simulink model "FMtestHarness"  (R2024b)
settings: Solver=VariableStepAuto  StartTime=0.0  StopTime=10.0  RelTol=1e-3  AbsTol=1e-3
model workspace: external: MAT-File VehicleharnessData.mat (data not in the file)
values from neighbouring files (symbols this model uses):
  VehicleHarn =     [VehicleharnessData.mat]
settings Model: DataDictionary=VTOLDynamicsData.sldd  Creator=saprasad  LastModifiedBy=jjha
settings SolverCC: AutoScaleAbsTol=off  AlgebraicLoopSolver=TrustRegion  MaxZcPerStep=1
settings DebuggingCC: UnconnectedInputMsg=warning  UnconnectedOutputMsg=warning  UnconnectedLineMsg=warning  SymbolicDimsDataTypeCodeGenerationDiagnostic=none
settings ModelReferenceCC: EnableRefExpFcnMdlSchedulingChecks=on
settings SFSimCC: CustomCodeUndefinedFunction=UseInterfaceOnly
settings RTWCC: GPUComputeCapability=3.5  DLArmComputeVersion=19.05
settings SimscapeCC: SimscapeLogType=all  SimscapeLogSimulationStatistics=on  SimscapeLogDataHistory=10000

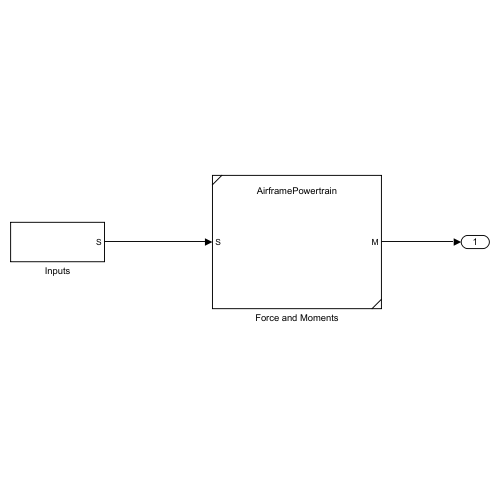
[thumbnail: Simulink's stored preview of the top-level diagram]
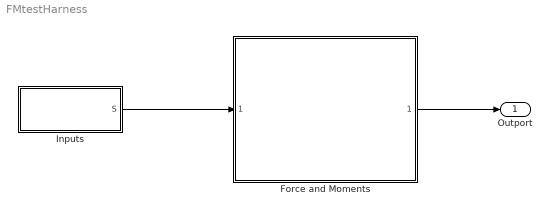
== system FMtestHarness ==
  Force and Moments : Subsystem  ReferencedSubsystem=AirframePowertrain
  Inputs : Subsystem
  Outport : Outport
  wires:
  Force and Moments/1 -> Outport/1
  Inputs/1(S) -> Force and Moments/1

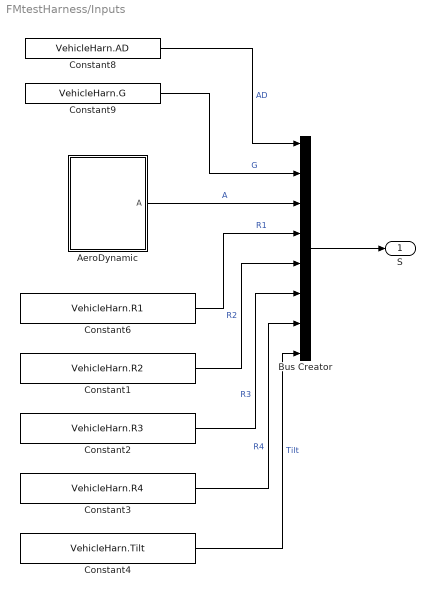
== system FMtestHarness/Inputs ==
  AeroDynamic : Subsystem
  Bus Creator : BusCreator  Inputs=8
  Constant1 : Constant  Value=VehicleHarn.R2  OutDataTypeStr=Bus: Vehicle_R2
  Constant2 : Constant  Value=VehicleHarn.R3  OutDataTypeStr=Bus: Vehicle_R3
  Constant3 : Constant  Value=VehicleHarn.R4  OutDataTypeStr=Bus: Vehicle_R4
  Constant4 : Constant  Value=VehicleHarn.Tilt  OutDataTypeStr=Bus: Vehicle_Tilt
  Constant6 : Constant  Value=VehicleHarn.R1  OutDataTypeStr=Bus: Vehicle_R1
  Constant8 : Constant  Value=VehicleHarn.AD  OutDataTypeStr=Bus: Vehicle_AD
  Constant9 : Constant  Value=VehicleHarn.G  OutDataTypeStr=Bus: Vehicle_G
  S : Outport
  wires:
  Constant8/1 -> Bus Creator/1  "AD"
  Bus Creator/1 -> S/1
  AeroDynamic/1(A) -> Bus Creator/3  "A"
  Constant9/1 -> Bus Creator/2  "G"
  Constant6/1 -> Bus Creator/4  "R1"
  Constant1/1 -> Bus Creator/5  "R2"
  Constant2/1 -> Bus Creator/6  "R3"
  Constant3/1 -> Bus Creator/7  "R4"
  Constant4/1 -> Bus Creator/8  "Tilt"

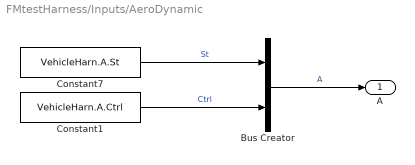
== system FMtestHarness/Inputs/AeroDynamic ==
  Bus Creator : BusCreator  Inputs=2
  Constant1 : Constant  Value=VehicleHarn.A.Ctrl  OutDataTypeStr=Bus: Vehicle_A_Ctrl
  Constant7 : Constant  Value=VehicleHarn.A.St  OutDataTypeStr=Bus: Vehicle_A_St
  A : Outport
  wires:
  Constant7/1 -> Bus Creator/1  "St"
  Bus Creator/1 -> A/1  "A"
  Constant1/1 -> Bus Creator/2  "Ctrl"
